simulink model "SPWMr2019"  (R2019b)
settings: Solver=ode1  StartTime=0.0  StopTime=2  FixedStep=1e-5  RelTol=1e-3
InitFcn:
  | %T=0.0000071
  | T = (1e-5)/2
  | 
  | flux=0.2068
undefined symbols (not defined in the file or in its folder): B, J, Kiq, Kiw, Kpq, Kpw, Lambda_m, Ld, Lq, P, Rs, Vdc
libraries: powerlib_meascontrol x3, modelsimlib x1
settings Model: Creator=samfi  LastModifiedBy=kanth

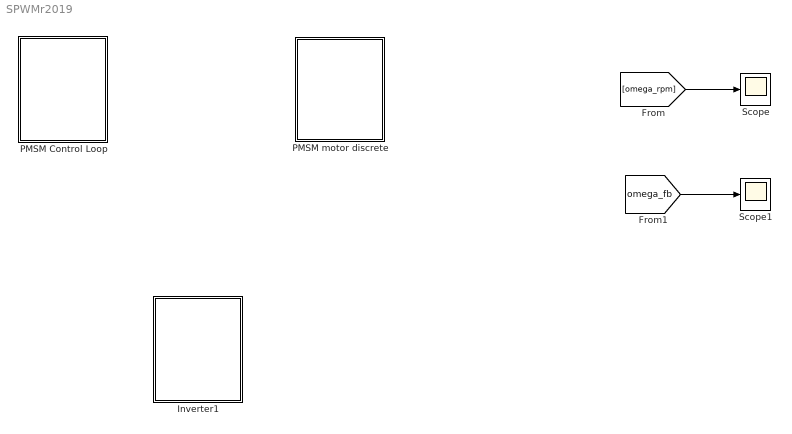
== system SPWMr2019 ==
  Inverter1 : Subsystem
  PMSM Control Loop : Subsystem
  PMSM motor discrete : Subsystem
  Scope : Scope
  Scope1 : Scope
  wires:
  [omega_rpm] -> Scope/1
  [omega_fb] -> Scope1/1

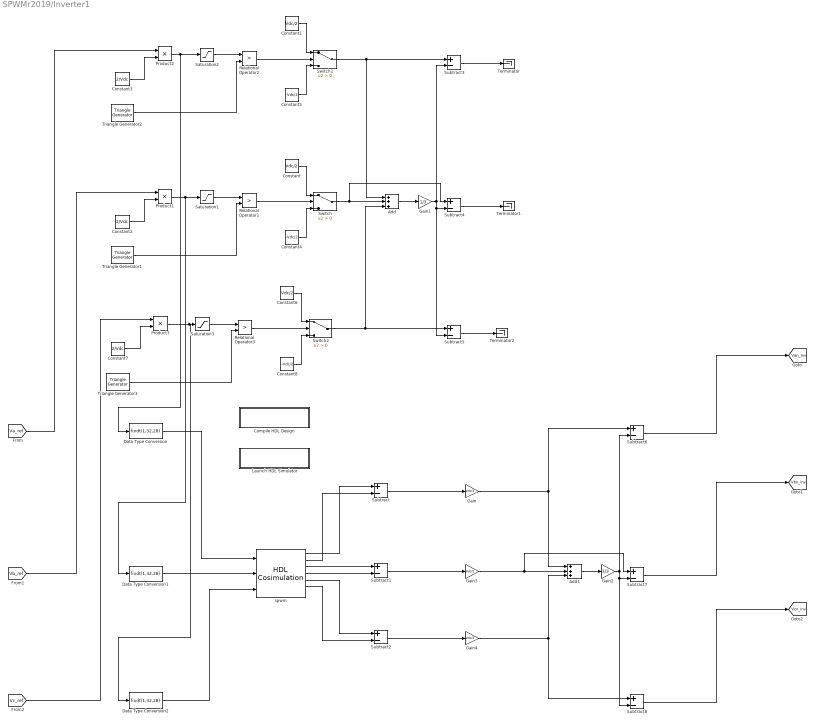
== system SPWMr2019/Inverter1 ==
  Add : Sum  Inputs=+++
  Add1 : Sum  Inputs=+++
  Compile HDL Design : Subsystem
      settings: OpenFcn=eval('compile_hdl_design_spwm');
      mask Display: disp(['Double-Click to' char(10) 'compile HDL files'])
  Constant : Constant  Value=Vdc/2
  Constant1 : Constant  Value=Vdc/2
  Constant2 : Constant  Value=2/Vdc
  Constant3 : Constant  Value=2/Vdc
  Constant4 : Constant  Value=-Vdc/2
  Constant5 : Constant  Value=-Vdc/2
  Constant6 : Constant  Value=Vdc/2
  Constant7 : Constant  Value=2/Vdc
  Constant8 : Constant  Value=-Vdc/2
  Data Type Conversion : DataTypeConversion  OutDataTypeStr=fixdt(1,32,28)
  Data Type Conversion1 : DataTypeConversion  OutDataTypeStr=fixdt(1,32,28)
  Data Type Conversion2 : DataTypeConversion  OutDataTypeStr=fixdt(1,32,28)
  Gain : Gain  Gain=Vdc/2  ParamDataTypeStr=double  OutDataTypeStr=double
  Gain1 : Gain  Gain=1/3
  Gain2 : Gain  Gain=1/3
  Gain3 : Gain  Gain=Vdc/2  ParamDataTypeStr=double  OutDataTypeStr=double
  Gain4 : Gain  Gain=Vdc/2  ParamDataTypeStr=double  OutDataTypeStr=double
  Launch HDL Simulator : Subsystem
      settings: OpenFcn=eval('launch_hdl_simulator_spwm');
      mask Display: disp(['Double-Click to' char(10) 'launch HDL simulator'])
  Product1 : Product
  Product2 : Product
  Product3 : Product
  Relational Operator1 : RelationalOperator  Operator=>  OutDataTypeStr=boolean  RndMeth=Simplest
  Relational Operator2 : RelationalOperator  Operator=>  OutDataTypeStr=boolean  RndMeth=Simplest
  Relational Operator3 : RelationalOperator  Operator=>  OutDataTypeStr=boolean  RndMeth=Simplest
  Saturation1 : Saturate  UpperLimit=0.9  LowerLimit=-0.9
  Saturation2 : Saturate  UpperLimit=0.9  LowerLimit=-0.9
  Saturation3 : Saturate  UpperLimit=0.9  LowerLimit=-0.9
  Subtract : Sum  Inputs=+-  AccumDataTypeStr=double  OutDataTypeStr=double
  Subtract1 : Sum  Inputs=+-  AccumDataTypeStr=double  OutDataTypeStr=double
  Subtract2 : Sum  Inputs=+-  AccumDataTypeStr=double  OutDataTypeStr=double
  Subtract{3..8} (6 alike) : Sum  Inputs=+-
  Switch : Switch  Criteria=u2 > Threshold
  Switch1 : Switch  Criteria=u2 > Threshold
  Switch2 : Switch  Criteria=u2 > Threshold
  Terminator : Terminator
  Terminator1 : Terminator
  Terminator2 : Terminator
  Triangle Generator1 : powerlib_meascontrol/Pulse & Signal Generators/Triangle Generator  Freq=1e4  Phase=0  Ts=0
  Triangle Generator2 : powerlib_meascontrol/Pulse & Signal Generators/Triangle Generator  Freq=1e4  Phase=0  Ts=0
  Triangle Generator3 : powerlib_meascontrol/Pulse & Signal Generators/Triangle Generator  Freq=1e4  Phase=0  Ts=0
  spwm : modelsimlib/HDL Cosimulation  PortPaths=/spwm/x;/spwm/y;/spwm/z;/spwm/Sau;/spwm/Sal;/spwm/Sbu;/spwm/Sbl;/spwm/Scu;/spwm/Scl;/spwm/out;  PortModes=[1 1 1 2 2 2 2 2 2 2 ]  PortTimes=[-1,-1,-1,1e-5,1e-5,1e-5,1e-5,1e-5,1e-5,1e-5]  PortSigns=[-1,-1,-1,0,0,0,0,0,0,1,]  PortFracLengths=[0,0,0,0,0,0,0,0,0,28]  CommLocal=on  CommSharedMemory=on  CommPortNumber=4449  CommShowInfo=on  ClockModes=[]  ClockTimes=[]  TclPreSimCommand=|  TclPostSimCommand=|  TimingMode=s  TimingScaleFactor=1  idxCellArray={'UNUSED_VAR'}  CosimBypass=Full Simulation  AllowDirectFeedthrough=on  ProductName=EDA Simulator Link MQ  RunAutoTimescale=off  HdlClocks=/spwm/clk 10 ns;  PreRunTime=10  PreRunTimeUnit=ns
      TclPreSimCommand=|
      | force /spwm/clk 0 0 ns, 1 5 ns -repeat 10 ns;
      | force /spwm/res 1 0 ns, 0 8 ns;
      TclPostSimCommand=|
      | noforce /spwm/clk;
      | noforce /spwm/res;
      | puts "done";
      settings: SourceProductBaseCode=ES
  tag scope: Van_inv=global, Vbn_inv=global, Vcn_inv=global
  wires:
  Subtract/1 -> Gain/1
  Subtract1/1 -> Gain3/1
  Subtract2/1 -> Gain4/1
  Add/1 -> Gain1/1
  Constant7/1 -> Product3/2
  [Vb_ref] -> Product1/1
  Product2/1 -> Data Type Conversion/1, Saturation2/1
  Constant8/1 -> Switch2/3
  Triangle Generator3/1 -> Relational Operator3/2
  [Vc_ref] -> Product3/1
  Constant3/1 -> Product2/2
  Saturation2/1 -> Relational Operator2/1
  Triangle Generator2/1 -> Relational Operator2/2
  Constant6/1 -> Switch2/1
  Switch1/1 -> Subtract3/1, Add/1
  Switch2/1 -> Subtract5/1, Add/3
  Product3/1 -> Data Type Conversion2/1, Saturation3/1
  Constant4/1 -> Switch/3
  Relational Operator2/1 -> Switch1/2
  Constant5/1 -> Switch1/3
  Triangle Generator1/1 -> Relational Operator1/2
  [Va_ref] -> Product2/1
  Constant/1 -> Switch/1
  Gain1/1 -> Subtract5/2, Subtract4/2, Subtract3/2
  Constant1/1 -> Switch1/1
  Saturation3/1 -> Relational Operator3/1
  Relational Operator1/1 -> Switch/2
  Relational Operator3/1 -> Switch2/2
  Switch/1 -> Subtract4/1, Add/2
  Constant2/1 -> Product1/2
  Saturation1/1 -> Relational Operator1/1
  Product1/1 -> Saturation1/1, Data Type Conversion1/1
  Data Type Conversion1/1 -> spwm/2
  Data Type Conversion/1 -> spwm/1
  Data Type Conversion2/1 -> spwm/3
  spwm/1 -> Subtract/1
  spwm/2 -> Subtract/2
  spwm/3 -> Subtract1/1
  spwm/4 -> Subtract1/2
  spwm/5 -> Subtract2/1
  spwm/6 -> Subtract2/2
  Subtract3/1 -> Terminator/1
  Subtract4/1 -> Terminator1/1
  Subtract5/1 -> Terminator2/1
  Subtract7/1 -> [Vbn_inv]
  Subtract8/1 -> [Vcn_inv]
  Gain3/1 -> Subtract7/1, Add1/2
  Gain2/1 -> Subtract8/2, Subtract7/2, Subtract6/2
  Gain4/1 -> Subtract8/1, Add1/3
  Gain/1 -> Subtract6/1, Add1/1
  Add1/1 -> Gain2/1
  Subtract6/1 -> [Van_inv]

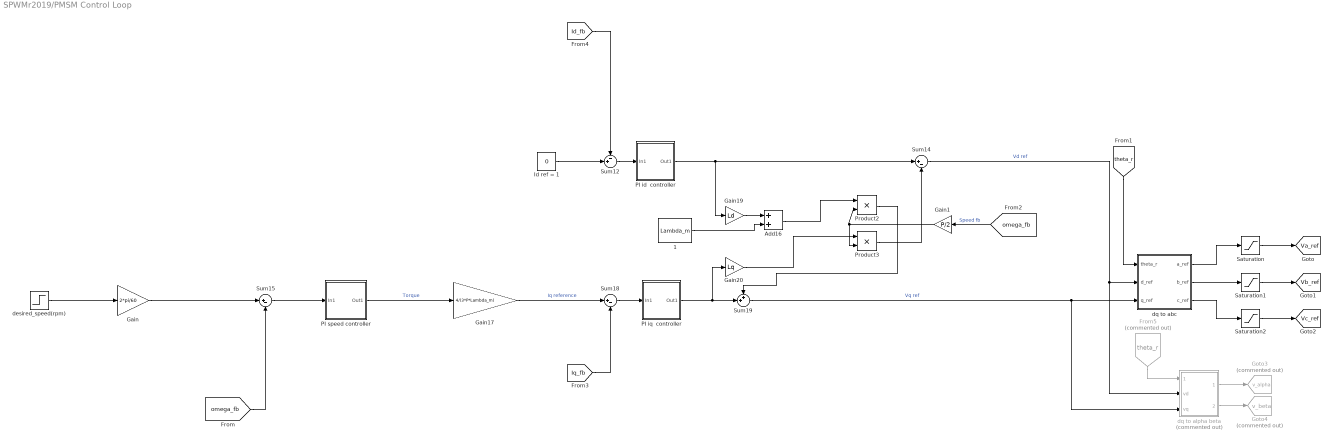
== system SPWMr2019/PMSM Control Loop ==
  " 1" : Constant  Value=Lambda_m  SampleTime=1e-4
  Add16 : Sum
  From5 : From  Commented=on  GotoTag=theta_r  TagVisibility=global
  Gain : Gain  Gain=2*pi/60
  Gain1 : Gain  Gain=P/2
  Gain17 : Gain  Gain=4/(3*P*Lambda_m)
  Gain19 : Gain  Gain=Ld
  Gain20 : Gain  Gain=Lq
  Goto3 : Goto  Commented=on  GotoTag=v_alpha  TagVisibility=global
  Goto4 : Goto  Commented=on  GotoTag=v_beta  TagVisibility=global
  Id ref = 1 : Constant  Value=0  SampleTime=1e-4
  PI id  controller : Subsystem
  PI iq  controller : Subsystem
  PI speed controller : Subsystem
  Product2 : Product
  Product3 : Product
  Saturation : Saturate  UpperLimit=200  LowerLimit=-200
  Saturation1 : Saturate  UpperLimit=200  LowerLimit=-200
  Saturation2 : Saturate  UpperLimit=200  LowerLimit=-200
  Sum12 : Sum  Inputs=-+|
  Sum14 : Sum  Inputs=|+-
  Sum15 : Sum  Inputs=|+-
  Sum18 : Sum  Inputs=|+-
  Sum19 : Sum  Inputs=++|
  desired_speed(rpm) : Step  Time=0.25  After=400  SampleTime=1e-4
  dq to abc : Subsystem
  dq to alpha beta : Subsystem  Commented=on
  tag scope: Va_ref=global, Vb_ref=global, Vc_ref=global
  wires:
  Product2/1 -> Sum19/1
  Add16/1 -> Product2/1
  Gain20/1 -> Product3/1
  Product3/1 -> Sum14/2
  Id ref = 1/1 -> Sum12/2
  PI iq  controller/1(Out1) -> Gain20/1, Sum19/2
  PI id  controller/1(Out1) -> Gain19/1, Sum14/1
  Sum14/1 -> dq to alpha beta/2(vd), dq to abc/2(d_ref)  "Vd ref"
  Gain19/1 -> Add16/1
  Sum18/1 -> PI iq  controller/1(In1)
  " 1"/1 -> Add16/2
  Gain17/1 -> Sum18/1  "Iq reference"
  Sum19/1 -> dq to alpha beta/3(vq), dq to abc/3(q_ref)  "Vq ref"
  [omega_fb] -> Sum15/2
  [theta_r] -> dq to abc/1(theta_r)
  [Iq_fb] -> Sum18/2
  [Id_fb] -> Sum12/1
  Saturation/1 -> [Va_ref]
  Saturation1/1 -> [Vb_ref]
  Saturation2/1 -> [Vc_ref]
  dq to abc/3(c_ref) -> Saturation2/1
  dq to abc/1(a_ref) -> Saturation/1
  dq to abc/2(b_ref) -> Saturation1/1
  Gain/1 -> Sum15/1
  [omega_fb] -> Gain1/1  "Speed fb"
  Gain1/1 -> Product3/2, Product2/2
  Sum12/1 -> PI id  controller/1(In1)
  Sum15/1 -> PI speed controller/1(In1)
  PI speed controller/1(Out1) -> Gain17/1  "Torque"
  dq to alpha beta/1(valpha) -> Goto3/1
  dq to alpha beta/2(vbeta) -> Goto4/1
  From5/1 -> dq to alpha beta/1(theta_r)
  desired_speed(rpm)/1 -> Gain/1

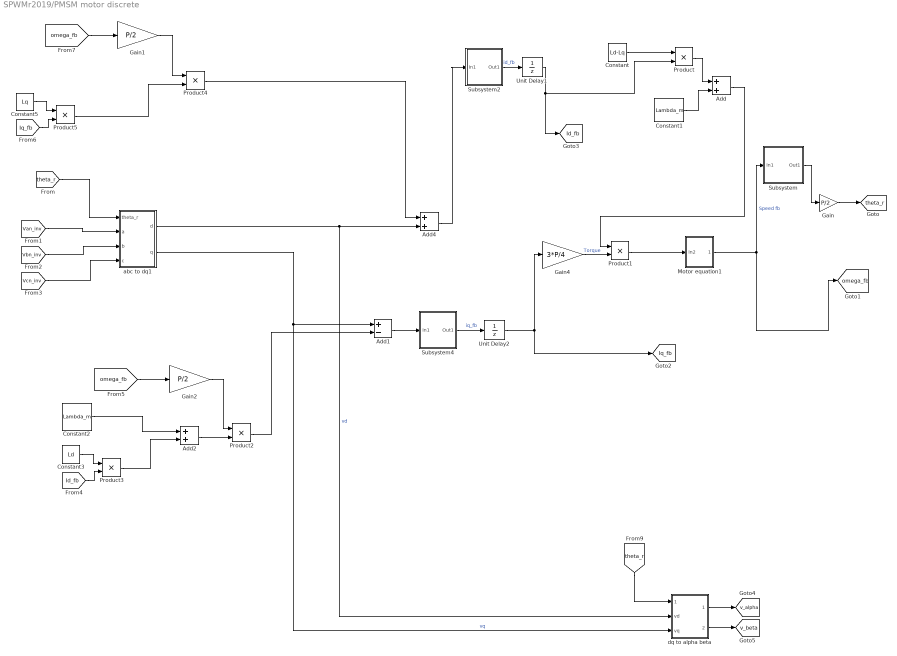
== system SPWMr2019/PMSM motor discrete ==
  Add : Sum
  Add1 : Sum  Inputs=+-
  Add2 : Sum
  Add4 : Sum
  Constant : Constant  Value=Ld-Lq  SampleTime=1e-4
  Constant1 : Constant  Value=Lambda_m  SampleTime=1e-4
  Constant2 : Constant  Value=Lambda_m  SampleTime=1e-4
  Constant3 : Constant  Value=Ld  SampleTime=1e-4
  Constant5 : Constant  Value=Lq  SampleTime=1e-4
  Gain : Gain  Gain=P/2
  Gain1 : Gain  Gain=P/2
  Gain2 : Gain  Gain=P/2
  Gain4 : Gain  Gain=3*P/4
  Motor equation1 : Subsystem
  Product{,1..5} (6 alike) : Product
  Subsystem : Subsystem
  Subsystem2 : Subsystem
  Subsystem4 : Subsystem
  Unit Delay1 : UnitDelay  SampleTime=-1  HasFrameUpgradeWarning=on
  Unit Delay2 : UnitDelay  SampleTime=-1  HasFrameUpgradeWarning=on
  abc to dq1 : Subsystem
  dq to alpha beta : Subsystem
  tag scope: Id_fb=global, Iq_fb=global, omega_fb=global, theta_r=global, v_alpha=global, v_beta=global
  wires:
  Subsystem4/1(Out1) -> Unit Delay2/1  "iq_fb"
  [Vbn_inv] -> abc to dq1/3(b)
  Motor equation1/1(Out1) -> [omega_fb], Subsystem/1(In1)  "Speed fb"
  [Van_inv] -> abc to dq1/2(a)
  [Vcn_inv] -> abc to dq1/4(c)
  Subsystem2/1(Out1) -> Unit Delay1/1  "id_fb"
  Product1/1 -> Motor equation1/1(In2)
  Constant/1 -> Product/1
  Product/1 -> Add/1
  Constant1/1 -> Add/2
  Gain4/1 -> Product1/2  "Torque"
  Add/1 -> Product1/1
  Subsystem/1(Out1) -> Gain/1
  Gain/1 -> [theta_r]
  abc to dq1/2(q) -> dq to alpha beta/3(vq), Add1/1  "vq"
  Product2/1 -> Add1/2
  [omega_fb] -> Gain2/1
  Constant3/1 -> Product3/1
  [Id_fb] -> Product3/2
  Product3/1 -> Add2/2
  Constant2/1 -> Add2/1
  Add2/1 -> Product2/2
  [Iq_fb] -> Product5/2
  Product5/1 -> Product4/2
  Constant5/1 -> Product5/1
  abc to dq1/1(d) -> dq to alpha beta/2(vd), Add4/2  "vd"
  Product4/1 -> Add4/1
  [omega_fb] -> Gain1/1
  Gain1/1 -> Product4/1
  Gain2/1 -> Product2/1
  dq to alpha beta/1(valpha) -> [v_alpha]
  dq to alpha beta/2(vbeta) -> [v_beta]
  [theta_r] -> abc to dq1/1(theta_r)
  [theta_r] -> dq to alpha beta/1(theta_r)
  Add4/1 -> Subsystem2/1(In1)
  Add1/1 -> Subsystem4/1(In1)
  Unit Delay1/1 -> [Id_fb], Product/2
  Unit Delay2/1 -> Gain4/1, [Iq_fb]

== system SPWMr2019/Inverter1/Compile HDL Design ==

== system SPWMr2019/Inverter1/Launch HDL Simulator ==

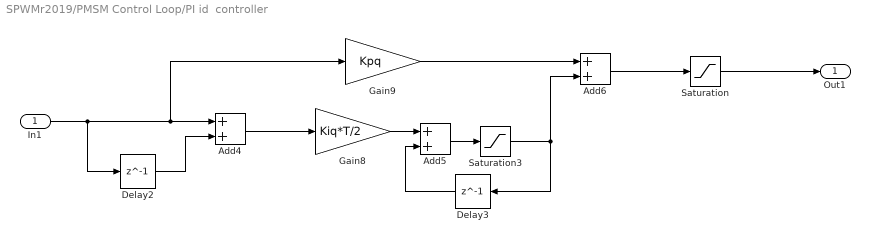
== system SPWMr2019/PMSM Control Loop/PI id  controller ==
  In1 : Inport
  Add4 : Sum
  Add5 : Sum
  Add6 : Sum
  Delay2 : Delay  DelayLength=1
  Delay3 : Delay  DelayLength=1
  Gain8 : Gain  Gain=Kiq*T/2
  Gain9 : Gain  Gain=Kpq
  Saturation : Saturate  UpperLimit=220  LowerLimit=-220
  Saturation3 : Saturate  UpperLimit=200  LowerLimit=-200
  Out1 : Outport
  wires:
  Gain8/1 -> Add5/1
  Delay2/1 -> Add4/2
  Add5/1 -> Saturation3/1
  Add4/1 -> Gain8/1
  Saturation3/1 -> Delay3/1, Add6/2
  In1/1 -> Add4/1, Gain9/1, Delay2/1
  Gain9/1 -> Add6/1
  Delay3/1 -> Add5/2
  Add6/1 -> Saturation/1
  Saturation/1 -> Out1/1

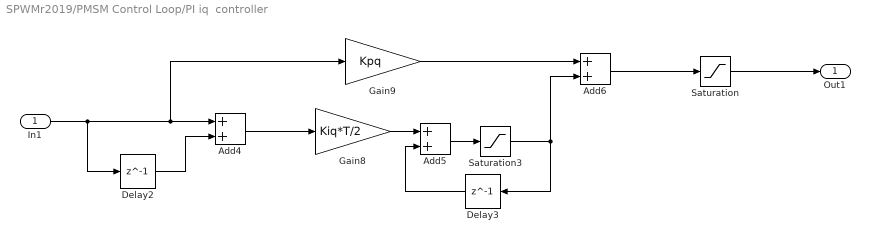
== system SPWMr2019/PMSM Control Loop/PI iq  controller ==
  In1 : Inport
  Add4 : Sum
  Add5 : Sum
  Add6 : Sum
  Delay2 : Delay  DelayLength=1
  Delay3 : Delay  DelayLength=1
  Gain8 : Gain  Gain=Kiq*T/2
  Gain9 : Gain  Gain=Kpq
  Saturation : Saturate  UpperLimit=220  LowerLimit=-220
  Saturation3 : Saturate  UpperLimit=200  LowerLimit=-200
  Out1 : Outport
  wires:
  Delay3/1 -> Add5/2
  Gain9/1 -> Add6/1
  In1/1 -> Delay2/1, Gain9/1, Add4/1
  Saturation3/1 -> Add6/2, Delay3/1
  Add4/1 -> Gain8/1
  Add5/1 -> Saturation3/1
  Delay2/1 -> Add4/2
  Gain8/1 -> Add5/1
  Add6/1 -> Saturation/1
  Saturation/1 -> Out1/1

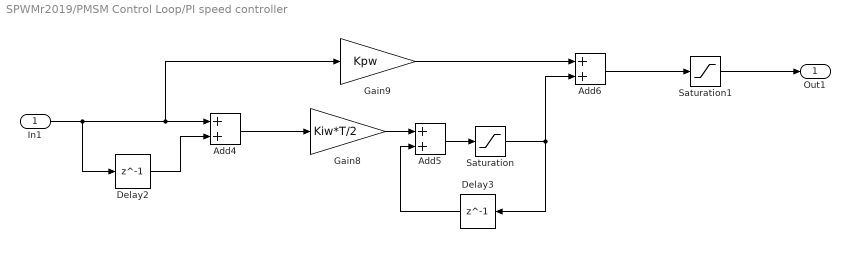
== system SPWMr2019/PMSM Control Loop/PI speed controller ==
  In1 : Inport
  Add4 : Sum
  Add5 : Sum
  Add6 : Sum
  Delay2 : Delay  DelayLength=1
  Delay3 : Delay  DelayLength=1
  Gain8 : Gain  Gain=Kiw*T/2
  Gain9 : Gain  Gain=Kpw
  Saturation : Saturate  UpperLimit=10  LowerLimit=-10
  Saturation1 : Saturate  UpperLimit=10  LowerLimit=-10
  Out1 : Outport
  wires:
  Gain9/1 -> Add6/1
  Delay2/1 -> Add4/2
  Gain8/1 -> Add5/1
  Add5/1 -> Saturation/1
  In1/1 -> Delay2/1, Gain9/1, Add4/1
  Saturation/1 -> Add6/2, Delay3/1
  Add4/1 -> Gain8/1
  Delay3/1 -> Add5/2
  Add6/1 -> Saturation1/1
  Saturation1/1 -> Out1/1

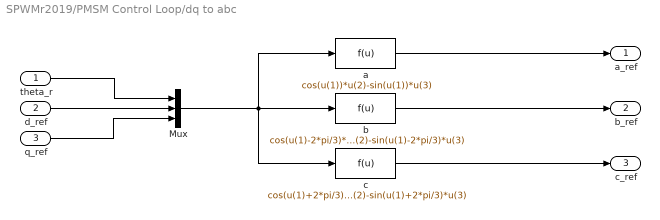
== system SPWMr2019/PMSM Control Loop/dq to abc ==
  theta_r : Inport
  d_ref : Inport  Port=2
  q_ref : Inport  Port=3
  Mux : Mux  Inputs=3
  a : Fcn  Expr=cos(u(1))*u(2)-sin(u(1))*u(3)
  b : Fcn  Expr=cos(u(1)-2*pi/3)*u(2)-sin(u(1)-2*pi/3)*u(3)
  c : Fcn  Expr=cos(u(1)+2*pi/3)*u(2)-sin(u(1)+2*pi/3)*u(3)
  a_ref : Outport
  b_ref : Outport  Port=2
  c_ref : Outport  Port=3
  wires:
  d_ref/1 -> Mux/2
  Mux/1 -> c/1, b/1, a/1
  c/1 -> c_ref/1
  theta_r/1 -> Mux/1
  b/1 -> b_ref/1
  a/1 -> a_ref/1
  q_ref/1 -> Mux/3

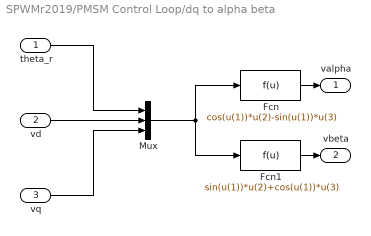
== system SPWMr2019/PMSM Control Loop/dq to alpha beta ==
  theta_r : Inport
  vd : Inport  Port=2
  vq : Inport  Port=3
  Fcn : Fcn  Expr=cos(u(1))*u(2)-sin(u(1))*u(3)
  Fcn1 : Fcn  Expr=sin(u(1))*u(2)+cos(u(1))*u(3)
  Mux : Mux  Inputs=3
  valpha : Outport
  vbeta : Outport  Port=2
  wires:
  Mux/1 -> Fcn/1, Fcn1/1
  vq/1 -> Mux/3
  theta_r/1 -> Mux/1
  Fcn1/1 -> vbeta/1
  vd/1 -> Mux/2
  Fcn/1 -> valpha/1

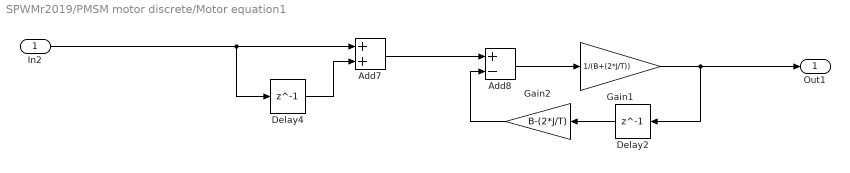
== system SPWMr2019/PMSM motor discrete/Motor equation1 ==
  In2 : Inport
  Add7 : Sum
  Add8 : Sum  Inputs=+-
  Delay2 : Delay  DelayLength=1
  Delay4 : Delay  DelayLength=1
  Gain1 : Gain  Gain=1/(B+(2*J/T))
  Gain2 : Gain  Gain=B-(2*J/T)
  Out1 : Outport
  wires:
  Add7/1 -> Add8/1
  Gain1/1 -> Out1/1, Delay2/1
  Delay2/1 -> Gain2/1
  Add8/1 -> Gain1/1
  Gain2/1 -> Add8/2
  In2/1 -> Delay4/1, Add7/1
  Delay4/1 -> Add7/2

== system SPWMr2019/PMSM motor discrete/Subsystem ==
  In1 : Inport
  Add1 : Sum
  Add2 : Sum
  Delay1 : Delay  DelayLength=1
  Delay4 : Delay  DelayLength=1
  Gain : Gain  Gain=T/2
  Out1 : Outport
  wires:
  In1/1 -> Delay4/1, Add1/1
  Delay1/1 -> Add2/2
  Add2/1 -> Out1/1, Delay1/1
  Delay4/1 -> Add1/2
  Add1/1 -> Gain/1
  Gain/1 -> Add2/1

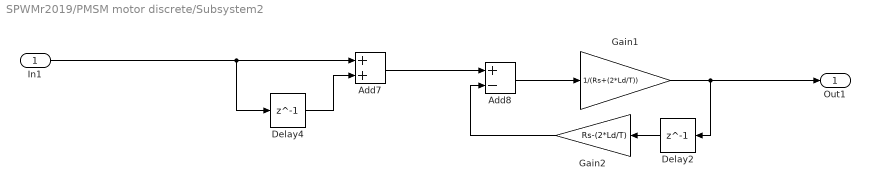
== system SPWMr2019/PMSM motor discrete/Subsystem2 ==
  In1 : Inport
  Add7 : Sum
  Add8 : Sum  Inputs=+-
  Delay2 : Delay  DelayLength=1
  Delay4 : Delay  DelayLength=1
  Gain1 : Gain  Gain=1/(Rs+(2*Ld/T))
  Gain2 : Gain  Gain=Rs-(2*Ld/T)
  Out1 : Outport
  wires:
  Add8/1 -> Gain1/1
  In1/1 -> Add7/1, Delay4/1
  Gain2/1 -> Add8/2
  Delay2/1 -> Gain2/1
  Delay4/1 -> Add7/2
  Add7/1 -> Add8/1
  Gain1/1 -> Out1/1, Delay2/1

== system SPWMr2019/PMSM motor discrete/Subsystem4 ==
  In1 : Inport
  Add7 : Sum
  Add8 : Sum  Inputs=+-
  Delay2 : Delay  DelayLength=1
  Delay4 : Delay  DelayLength=1
  Gain1 : Gain  Gain=1/(Rs+(2*Lq/T))
  Gain2 : Gain  Gain=Rs-(2*Lq/T)
  Out1 : Outport
  wires:
  Add8/1 -> Gain1/1
  Gain1/1 -> Delay2/1, Out1/1
  Add7/1 -> Add8/1
  Delay4/1 -> Add7/2
  Delay2/1 -> Gain2/1
  Gain2/1 -> Add8/2
  In1/1 -> Delay4/1, Add7/1

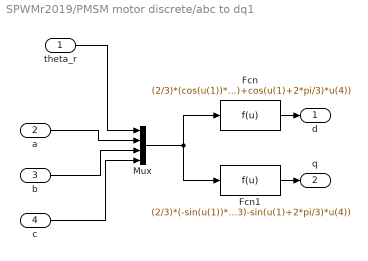
== system SPWMr2019/PMSM motor discrete/abc to dq1 ==
  theta_r : Inport
  a : Inport  Port=2
  b : Inport  Port=3
  c : Inport  Port=4
  Fcn : Fcn  Expr=(2/3)*(cos(u(1))*u(2)+cos(u(1)-2*pi/3)*u(3)+cos(u(1)+2*pi/3)*u(4))
  Fcn1 : Fcn  Expr=(2/3)*(-sin(u(1))*u(2)-sin(u(1)-2*pi/3)*u(3)-sin(u(1)+2*pi/3)*u(4))
  Mux : Mux
  d : Outport
  q : Outport  Port=2
  wires:
  a/1 -> Mux/2
  c/1 -> Mux/4
  theta_r/1 -> Mux/1
  Mux/1 -> Fcn/1, Fcn1/1
  b/1 -> Mux/3
  Fcn/1 -> d/1
  Fcn1/1 -> q/1

== system SPWMr2019/PMSM motor discrete/dq to alpha beta ==
  theta_r : Inport
  vd : Inport  Port=2
  vq : Inport  Port=3
  Fcn : Fcn  Expr=cos(u(1))*u(2)-sin(u(1))*u(3)
  Fcn1 : Fcn  Expr=sin(u(1))*u(2)+cos(u(1))*u(3)
  Mux : Mux  Inputs=3
  valpha : Outport
  vbeta : Outport  Port=2
  wires:
  Mux/1 -> Fcn/1, Fcn1/1
  vq/1 -> Mux/3
  theta_r/1 -> Mux/1
  Fcn1/1 -> vbeta/1
  vd/1 -> Mux/2
  Fcn/1 -> valpha/1
